simulink model "ITD_new"  (Simulink 7.9)
settings: Solver=ode45  StartTime=0.0  StopTime=1  FixedStep=0.001e-3  RelTol=1e-8  AbsTol=1e-11
values from neighbouring files (symbols this model uses):
  E_FB_EN2 = 1    [ITD_new_Sim.m]
  E_FB_EN3 = 0    [ITD_new_Sim.m]
  Etot1_const = 0e-9    (= 0)    [ITD_new_Sim.m]
  Etot1_rate = 100e-9    (= 1e-07)    [ITD_new_Sim.m]
  Etot2 = 10e-9    (= 1e-08)    [ITD_new_Sim.m]
  KD1 = 10e-9    (= 1e-08)    [ITD_new_Sim.m]
  KD2 = 50e-9    (= 5e-08)    [ITD_new_Sim.m]
  KD3 = 50e-9    (= 5e-08)    [ITD_new_Sim.m]
  kr2 = 100    [ITD_new_Sim.m]
  kr3 = 100    [ITD_new_Sim.m]
  n = 1    [ITD_new_Sim.m]
  r1 = 800    [ITD_new_Sim.m]
  r2 = 800    [ITD_new_Sim.m]
  S_FB_EN2 = 1    [ITD_new_Sim.m]
  S_FB_EN3 = 1    [ITD_new_Sim.m]
  Stot1 = Stot1_ss(i)    [ITD_new_Sim.m]
settings Model: Creator=lorenzo  LastModifiedBy=sswoo
settings SolverCC: ZeroCrossControl=DisableAll
settings DebuggingCC: FcnCallInpInsideContextMsg=Use local settings
settings GRTTargetCC: CombineOutputUpdateFcns=off  GRTInterface=on

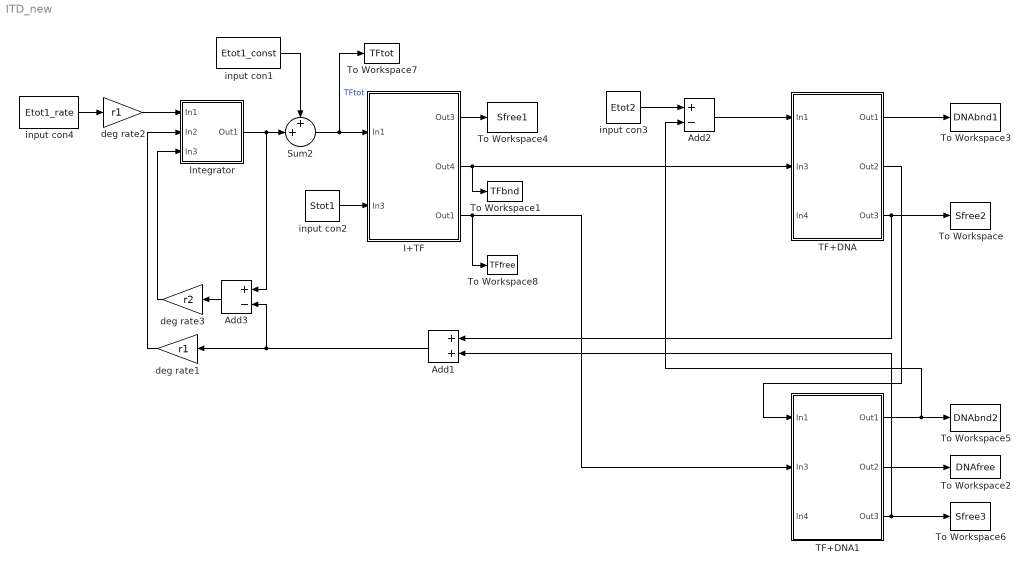
== system ITD_new ==
  Add1 : Sum
  Add2 : Sum  Inputs=+-
  Add3 : Sum  Inputs=+-
  I+TF : Subsystem
  Integrator : Subsystem
  Sum2 : Sum  Inputs=++|
  TF+DNA : Subsystem
  TF+DNA1 : Subsystem
  To Workspace : ToWorkspace  VariableName=Sfree2  SampleTime=-1  SaveFormat=Timeseries
  To Workspace1 : ToWorkspace  VariableName=TFbnd  SampleTime=-1  SaveFormat=Timeseries
  To Workspace2 : ToWorkspace  VariableName=DNAfree  SampleTime=-1  SaveFormat=Timeseries
  To Workspace3 : ToWorkspace  VariableName=DNAbnd1  SampleTime=-1  SaveFormat=Timeseries
  To Workspace4 : ToWorkspace  VariableName=Sfree1  SampleTime=-1  SaveFormat=Timeseries
  To Workspace5 : ToWorkspace  VariableName=DNAbnd2  SampleTime=-1  SaveFormat=Timeseries
  To Workspace6 : ToWorkspace  VariableName=Sfree3  SampleTime=-1  SaveFormat=Timeseries
  To Workspace7 : ToWorkspace  VariableName=TFtot  SampleTime=-1  SaveFormat=Timeseries
  To Workspace8 : ToWorkspace  VariableName=TFfree  SampleTime=-1  SaveFormat=Timeseries
  deg rate1 : Gain  Gain=r1
  deg rate2 : Gain  Gain=r1
  deg rate3 : Gain  Gain=r2
  input con1 : Constant  Value=Etot1_const
  input con2 : Constant  Value=Stot1
  input con3 : Constant  Value=Etot2
  input con4 : Constant  Value=Etot1_rate
  wires:
  input con2/1 -> I+TF/2(In3)
  TF+DNA/1(Out1) -> To Workspace3/1
  TF+DNA/2(Out2) -> TF+DNA1/1(In1)
  I+TF/1(Out3) -> To Workspace4/1
  I+TF/2(Out4) -> To Workspace1/1, TF+DNA/2(In3)
  I+TF/3(Out1) -> To Workspace8/1, TF+DNA1/2(In3)
  input con3/1 -> Add2/1
  Add2/1 -> TF+DNA/1(In1)
  TF+DNA1/1(Out1) -> Add2/2, To Workspace5/1
  TF+DNA1/2(Out2) -> To Workspace2/1
  TF+DNA/3(Out3) -> To Workspace/1, Add1/1
  TF+DNA1/3(Out3) -> To Workspace6/1, Add1/2
  Integrator/1(Out1) -> Sum2/2, Add3/1
  Sum2/1 -> I+TF/1(In1), To Workspace7/1  "TFtot"
  input con1/1 -> Sum2/1
  input con4/1 -> deg rate2/1
  Add1/1 -> Add3/2, deg rate1/1
  Add3/1 -> deg rate3/1
  deg rate1/1 -> Integrator/2(In2)
  deg rate2/1 -> Integrator/1(In1)
  deg rate3/1 -> Integrator/3(In3)

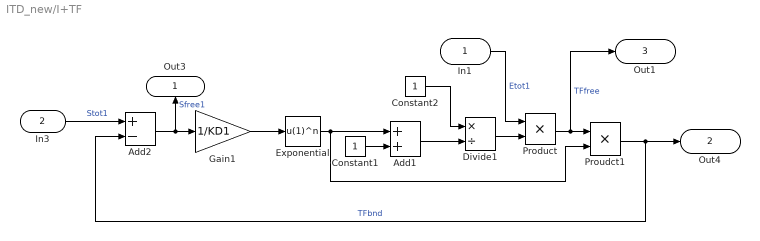
== system ITD_new/I+TF ==
  In1 : Inport
  In3 : Inport  Port=2
  Add1 : Sum
  Add2 : Sum  Inputs=+-
  Constant1 : Constant
  Constant2 : Constant
  Divide1 : Product  Inputs=*/
  Exponential : Fcn  Expr=u(1)^n
  Gain1 : Gain  Gain=1/KD1
  Product : Product  RndMeth=Zero
  Proudct1 : Product  RndMeth=Zero
  Out3 : Outport
  Out4 : Outport  Port=2
  Out1 : Outport  Port=3
  wires:
  Add2/1 -> Out3/1, Gain1/1  "Sfree1"
  In3/1 -> Add2/1  "Stot1"
  Gain1/1 -> Exponential/1
  Constant1/1 -> Add1/2
  Exponential/1 -> Add1/1, Proudct1/2
  Add1/1 -> Divide1/2
  Constant2/1 -> Divide1/1
  Divide1/1 -> Product/2
  In1/1 -> Product/1  "Etot1"
  Product/1 -> Out1/1, Proudct1/1  "TFfree"
  Proudct1/1 -> Out4/1, Add2/2  "TFbnd"

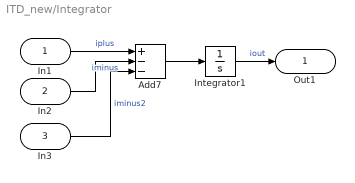
== system ITD_new/Integrator ==
  In1 : Inport
  In2 : Inport  Port=2
  In3 : Inport  Port=3
  Add7 : Sum  Inputs=+--
  Integrator1 : Integrator
  Out1 : Outport
  wires:
  Add7/1 -> Integrator1/1
  In1/1 -> Add7/1  "iplus"
  In2/1 -> Add7/2  "iminus"
  Integrator1/1 -> Out1/1  "iout"
  In3/1 -> Add7/3  "iminus2"

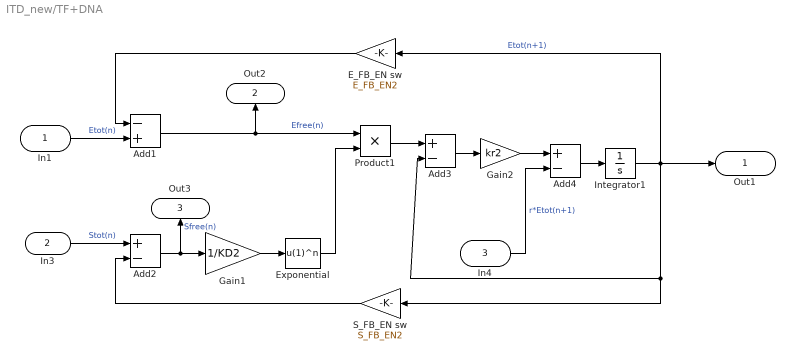
== system ITD_new/TF+DNA ==
  In1 : Inport
  In3 : Inport  Port=2
  In4 : Inport  Port=3
  Add1 : Sum  Inputs=-+
  Add2 : Sum  Inputs=+-
  Add3 : Sum  Inputs=+-
  Add4 : Sum  Inputs=+-
  E_FB_EN sw : Gain  Gain=E_FB_EN2
  Exponential : Fcn  Expr=u(1)^n
  Gain1 : Gain  Gain=1/KD2
  Gain2 : Gain  Gain=kr2
  Integrator1 : Integrator
  Product1 : Product  RndMeth=Zero
  S_FB_EN sw : Gain  Gain=S_FB_EN2
  Out1 : Outport
  Out2 : Outport  Port=2
  Out3 : Outport  Port=3
  wires:
  Add4/1 -> Integrator1/1
  In4/1 -> Add4/2  "r*Etot(n+1)"
  Gain2/1 -> Add4/1
  Integrator1/1 -> Out1/1, E_FB_EN sw/1, S_FB_EN sw/1, Add3/2  "Etot(n+1)"
  Exponential/1 -> Product1/2
  Gain1/1 -> Exponential/1
  In3/1 -> Add2/1  "Stot(n)"
  In1/1 -> Add1/2  "Etot(n)"
  Add1/1 -> Out2/1, Product1/1  "Efree(n)"
  Product1/1 -> Add3/1
  Add2/1 -> Out3/1, Gain1/1  "Sfree(n)"
  Add3/1 -> Gain2/1
  E_FB_EN sw/1 -> Add1/1
  S_FB_EN sw/1 -> Add2/2

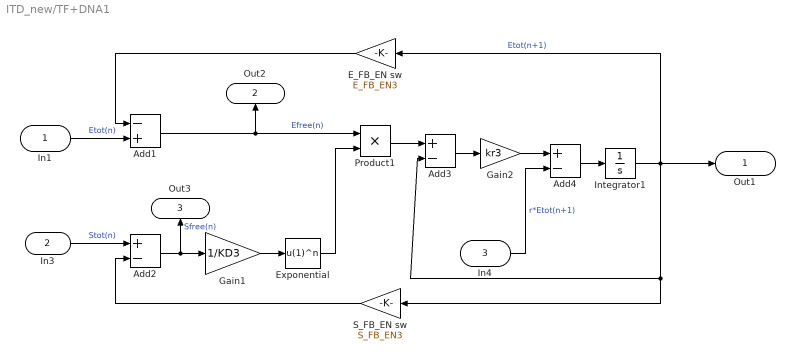
== system ITD_new/TF+DNA1 ==
  In1 : Inport
  In3 : Inport  Port=2
  In4 : Inport  Port=3
  Add1 : Sum  Inputs=-+
  Add2 : Sum  Inputs=+-
  Add3 : Sum  Inputs=+-
  Add4 : Sum  Inputs=+-
  E_FB_EN sw : Gain  Gain=E_FB_EN3
  Exponential : Fcn  Expr=u(1)^n
  Gain1 : Gain  Gain=1/KD3
  Gain2 : Gain  Gain=kr3
  Integrator1 : Integrator
  Product1 : Product  RndMeth=Zero
  S_FB_EN sw : Gain  Gain=S_FB_EN3
  Out1 : Outport
  Out2 : Outport  Port=2
  Out3 : Outport  Port=3
  wires:
  S_FB_EN sw/1 -> Add2/2
  E_FB_EN sw/1 -> Add1/1
  Add3/1 -> Gain2/1
  Add2/1 -> Gain1/1, Out3/1  "Sfree(n)"
  Product1/1 -> Add3/1
  Add1/1 -> Product1/1, Out2/1  "Efree(n)"
  In1/1 -> Add1/2  "Etot(n)"
  In3/1 -> Add2/1  "Stot(n)"
  Gain1/1 -> Exponential/1
  Exponential/1 -> Product1/2
  Integrator1/1 -> Add3/2, S_FB_EN sw/1, E_FB_EN sw/1, Out1/1  "Etot(n+1)"
  Gain2/1 -> Add4/1
  In4/1 -> Add4/2  "r*Etot(n+1)"
  Add4/1 -> Integrator1/1
